simulink model "Model_1"  (R2021a)
settings: Solver=VariableStepAuto  StartTime=0.0  StopTime=10.0  RelTol=1e-3
settings Model: Creator=DANI-TUF  LastModifiedBy=DANI-TUF

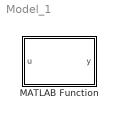
== system Model_1 ==
  MATLAB Function : MATLAB Function  Tag=thetadot  TreatAsAtomicUnit=on

== matlab function Model_1/MATLAB Function ==
  data: u input; y output
function y = fcn(u)



y = u;
